simulink model "arte"  (R2013b)
settings: Solver=ode45  StartTime=0.0  StopTime=10.0  RelTol=1e-3
undefined symbols (not defined in the file or in its folder): calan_lib, comp_addsub, sfp
libraries: xbsIndex_r4 x5087, casper_library_misc x65, casper_library_delays x48, dspsigops x32, xps_library x7, simulink x5
(part 8 of 43)

== system arte/bus_expand ==
  bus_in : Inport
  reinterpret{1..8} (8 alike) : xbsIndex_r4/Reinterpret  force_arith_type=on  arith_type="Signed  (2's comp)"  force_bin_pt=on  bin_pt=0  block_type=reinterpret
  slice1 : xbsIndex_r4/Slice  nbits=4  boolean_output=off  mode=Upper Bit Location + Width  bit1=-28  base1=MSB of Input  bit0=0  base0=LSB of Input  dbl_ovrd=off  block_type=slice
  slice2 : xbsIndex_r4/Slice  nbits=4  boolean_output=off  mode=Upper Bit Location + Width  bit1=-24  base1=MSB of Input  bit0=0  base0=LSB of Input  dbl_ovrd=off  block_type=slice
  slice3 : xbsIndex_r4/Slice  nbits=4  boolean_output=off  mode=Upper Bit Location + Width  bit1=-20  base1=MSB of Input  bit0=0  base0=LSB of Input  dbl_ovrd=off  block_type=slice
  slice4 : xbsIndex_r4/Slice  nbits=4  boolean_output=off  mode=Upper Bit Location + Width  bit1=-16  base1=MSB of Input  bit0=0  base0=LSB of Input  dbl_ovrd=off  block_type=slice
  slice5 : xbsIndex_r4/Slice  nbits=4  boolean_output=off  mode=Upper Bit Location + Width  bit1=-12  base1=MSB of Input  bit0=0  base0=LSB of Input  dbl_ovrd=off  block_type=slice
  slice6 : xbsIndex_r4/Slice  nbits=4  boolean_output=off  mode=Upper Bit Location + Width  bit1=-8  base1=MSB of Input  bit0=0  base0=LSB of Input  dbl_ovrd=off  block_type=slice
  slice7 : xbsIndex_r4/Slice  nbits=4  boolean_output=off  mode=Upper Bit Location + Width  bit1=-4  base1=MSB of Input  bit0=0  base0=LSB of Input  dbl_ovrd=off  block_type=slice
  slice8 : xbsIndex_r4/Slice  nbits=4  boolean_output=off  mode=Upper Bit Location + Width  bit1=0  base1=MSB of Input  bit0=0  base0=LSB of Input  dbl_ovrd=off  block_type=slice
  msb_out8 : Outport
  out7 : Outport  Port=2
  out6 : Outport  Port=3
  out5 : Outport  Port=4
  out4 : Outport  Port=5
  out3 : Outport  Port=6
  out2 : Outport  Port=7
  lsb_out1 : Outport  Port=8
  wires:
  bus_in/1 -> slice8/1, slice7/1, slice6/1, slice5/1, slice4/1, slice3/1, slice2/1, slice1/1
  slice8/1 -> reinterpret8/1
  reinterpret8/1 -> msb_out8/1
  slice7/1 -> reinterpret7/1
  reinterpret7/1 -> out7/1
  slice6/1 -> reinterpret6/1
  reinterpret6/1 -> out6/1
  slice5/1 -> reinterpret5/1
  reinterpret5/1 -> out5/1
  slice4/1 -> reinterpret4/1
  reinterpret4/1 -> out4/1
  slice3/1 -> reinterpret3/1
  reinterpret3/1 -> out3/1
  slice2/1 -> reinterpret2/1
  reinterpret2/1 -> out2/1
  slice1/1 -> reinterpret1/1
  reinterpret1/1 -> lsb_out1/1

== system arte/complex_add ==
  ff0_ch0 : Inport
  fft1_ch0 : Inport  Port=2
  fft0_ch1 : Inport  Port=3
  fft1_ch1 : Inport  Port=4
  fft0_ch2 : Inport  Port=5
  fft1_ch2 : Inport  Port=6
  fft0_ch3 : Inport  Port=7
  fft1_ch3 : Inport  Port=8
  sync : Inport  Port=9
  comp_addsub : Subsystem  AncestorBlock=calan_lib/comp_addsub  mask(comp_addsub){addsub=Addition, n_bits_in=18, bin_pt_in=17, add_latency=2, n_bits_out=18, bin_pt_out=17, quantization=Truncate, overflow=Wrap}
      mask prompts: addsub "Addition/Subtraction"; n_bits_in "Bit Width"; bin_pt_in "Binary Point"; add_latency "Adder Latency"; n_bits_out "Bit Width"; bin_pt_out "BInary Point"
      mask help: Add or substract two complex numbers of the same length.
      mask init:
      | comp_addsub_init(gcb, ...
      |     'addsub', addsub, ...
      |     'n_bits_in', n_bits_in, ...
      |     'bin_pt_in', bin_pt_in, ...
      |     'n_bits_out', n_bits_out, ...
      |     'bin_pt_out', bin_pt_out, ...
      |     'quantization', quantization, ...
      |     'overflow', overflow, ...
      |     'add_latency', add_latency);
      settings: AttributesFormatString=|
      | 18_17 * 18_17 ==> 18_17
      | Truncate, Wrap
      mask TypeOptions addsub: Addition | Subtraction
      mask TypeOptions quantization: Truncate | Round  (unbiased: +/- Inf)
      mask TypeOptions overflow: Wrap | Saturate | Flag as error
      mask Display:
      | port_label('input', 1, 'a');
      | port_label('input', 2, 'b');
      | if strcmp(addsub, 'Addition')
      |     port_label('output', 1, 'a+b');
      | elseif strcmp(addsub, 'Subtraction')
      |     port_label('output', 1, 'a-b');
      | end
      | disp(['Z^-', num2str(add_latency)]);
  comp_addsub1 : Subsystem  AncestorBlock=calan_lib/comp_addsub  mask(comp_addsub){addsub=Addition, n_bits_in=18, bin_pt_in=17, add_latency=2, n_bits_out=18, bin_pt_out=17, quantization=Truncate, overflow=Wrap}
      mask prompts: addsub "Addition/Subtraction"; n_bits_in "Bit Width"; bin_pt_in "Binary Point"; add_latency "Adder Latency"; n_bits_out "Bit Width"; bin_pt_out "BInary Point"
      mask help: Add or substract two complex numbers of the same length.
      mask init: same as arte/complex_add/comp_addsub
      settings: AttributesFormatString=|
      | 18_17 * 18_17 ==> 18_17
      | Truncate, Wrap
      mask TypeOptions addsub: Addition | Subtraction
      mask TypeOptions quantization: Truncate | Round  (unbiased: +/- Inf)
      mask TypeOptions overflow: Wrap | Saturate | Flag as error
      mask Display:
      | port_label('input', 1, 'a');
      | port_label('input', 2, 'b');
      | if strcmp(addsub, 'Addition')
      |     port_label('output', 1, 'a+b');
      | elseif strcmp(addsub, 'Subtraction')
      |     port_label('output', 1, 'a-b');
      | end
      | disp(['Z^-', num2str(add_latency)]);
  comp_addsub3 : Subsystem  AncestorBlock=calan_lib/comp_addsub  mask(comp_addsub){addsub=Addition, n_bits_in=18, bin_pt_in=17, add_latency=2, n_bits_out=18, bin_pt_out=17, quantization=Truncate, overflow=Wrap}
      mask prompts: addsub "Addition/Subtraction"; n_bits_in "Bit Width"; bin_pt_in "Binary Point"; add_latency "Adder Latency"; n_bits_out "Bit Width"; bin_pt_out "BInary Point"
      mask help: Add or substract two complex numbers of the same length.
      mask init: same as arte/complex_add/comp_addsub
      settings: AttributesFormatString=|
      | 18_17 * 18_17 ==> 18_17
      | Truncate, Wrap
      mask TypeOptions addsub: Addition | Subtraction
      mask TypeOptions quantization: Truncate | Round  (unbiased: +/- Inf)
      mask TypeOptions overflow: Wrap | Saturate | Flag as error
      mask Display:
      | port_label('input', 1, 'a');
      | port_label('input', 2, 'b');
      | if strcmp(addsub, 'Addition')
      |     port_label('output', 1, 'a+b');
      | elseif strcmp(addsub, 'Subtraction')
      |     port_label('output', 1, 'a-b');
      | end
      | disp(['Z^-', num2str(add_latency)]);
  comp_addsub6 : Subsystem  AncestorBlock=calan_lib/comp_addsub  mask(comp_addsub){addsub=Addition, n_bits_in=18, bin_pt_in=17, add_latency=2, n_bits_out=18, bin_pt_out=17, quantization=Truncate, overflow=Wrap}
      mask prompts: addsub "Addition/Subtraction"; n_bits_in "Bit Width"; bin_pt_in "Binary Point"; add_latency "Adder Latency"; n_bits_out "Bit Width"; bin_pt_out "BInary Point"
      mask help: Add or substract two complex numbers of the same length.
      mask init: same as arte/complex_add/comp_addsub
      settings: AttributesFormatString=|
      | 18_17 * 18_17 ==> 18_17
      | Truncate, Wrap
      mask TypeOptions addsub: Addition | Subtraction
      mask TypeOptions quantization: Truncate | Round  (unbiased: +/- Inf)
      mask TypeOptions overflow: Wrap | Saturate | Flag as error
      mask Display:
      | port_label('input', 1, 'a');
      | port_label('input', 2, 'b');
      | if strcmp(addsub, 'Addition')
      |     port_label('output', 1, 'a+b');
      | elseif strcmp(addsub, 'Subtraction')
      |     port_label('output', 1, 'a-b');
      | end
      | disp(['Z^-', num2str(add_latency)]);
  pipeline4 : Subsystem  AncestorBlock=casper_library_delays/pipeline  mask(pipeline){latency=2}
      mask help:
      | An explicitly laid-out delay line to avoid mapping to SRL16s
      | for use in pipelining to help achieve timing closure.
      mask init:
      | pipeline_init(gcb,'latency',latency);
      settings: AttributesFormatString=Latency = %<latency>
      mask Display:
      | port_label('input', 1, 'd');
      | port_label('output', 1, 'q');
      | disp(['Z^-', num2str(latency)]);
  sync_out : Outport
  ch0 : Outport  Port=2
  ch1 : Outport  Port=3
  ch2 : Outport  Port=4
  ch3 : Outport  Port=5
  wires:
  ff0_ch0/1 -> comp_addsub/1(a)
  fft1_ch0/1 -> comp_addsub/2(b)
  fft0_ch1/1 -> comp_addsub1/1(a)
  fft1_ch1/1 -> comp_addsub1/2(b)
  fft0_ch2/1 -> comp_addsub3/1(a)
  comp_addsub3/1(out) -> ch2/1
  fft1_ch2/1 -> comp_addsub3/2(b)
  fft0_ch3/1 -> comp_addsub6/1(a)
  fft1_ch3/1 -> comp_addsub6/2(b)
  sync/1 -> pipeline4/1(d)
  pipeline4/1(q) -> sync_out/1
  comp_addsub/1(out) -> ch0/1
  comp_addsub6/1(out) -> ch3/1
  comp_addsub1/1(out) -> ch1/1

== system arte/concat_ ==
  In1 : Inport
  In2 : Inport  Port=2
  In3 : Inport  Port=3
  In4 : Inport  Port=4
  Concat : xbsIndex_r4/Concat  num_inputs=4  dbl_ovrd=off  block_type=concat
  Reinterpret{,1..3} (4 alike) : xbsIndex_r4/Reinterpret  force_arith_type=off  arith_type=Unsigned  force_bin_pt=on  bin_pt=0  block_type=reinterpret
  Out1 : Outport
  wires:
  In4/1 -> Reinterpret/1
  In2/1 -> Reinterpret2/1
  In3/1 -> Reinterpret1/1
  In1/1 -> Reinterpret3/1
  Concat/1 -> Out1/1
  Reinterpret/1 -> Concat/1
  Reinterpret1/1 -> Concat/2
  Reinterpret2/1 -> Concat/3
  Reinterpret3/1 -> Concat/4

== system arte/concat_order ==
  ch0 : Inport
  ch1 : Inport  Port=2
  ch2 : Inport  Port=3
  ch3 : Inport  Port=4
  Concat : xbsIndex_r4/Concat  num_inputs=4  dbl_ovrd=off  block_type=concat
  Out1 : Outport
  wires:
  Concat/1 -> Out1/1
  ch0/1 -> Concat/4
  ch1/1 -> Concat/3
  ch2/1 -> Concat/2
  ch3/1 -> Concat/1
